simulink model "final"  (R2020b)
settings: Solver=ode4  StartTime=0.0  StopTime=10.0  FixedStep=ts  RelTol=1e-3
settings Model: Creator=auralius  LastModifiedBy=rishavgoenka
settings DataIOCC: LimitDataPoints=on  SaveFormat=Array  ReturnWorkspaceOutputs=off
settings OptimizationCC: BlockReduction=off  BooleanDataType=off  LifeSpan=inf
settings DebuggingCC: SaveWithParameterizedLinksMsg=none  UnderspecifiedInitializationDetection=Classic  MergeDetectMultiDrivingBlocksExec=none  SignalResolutionControl=TryResolveAllWithWarning  SFUnexpectedBacktrackingDiag=warning  SFNoUnconditionalDefaultTransitionDiag=warning  SFExecutionAtInitializationDiag=none  ArithmeticOperatorsInVariantConditions=warning
settings HardwareCC: ProdBitPerPointer=32  ProdBitPerSizeT=32  ProdBitPerPtrDiffT=32  ProdLargestAtomicFloat=None  ProdIntDivRoundTo=Undefined  ProdEndianess=Unspecified  ProdWordSize=32  ProdHWDeviceType=32-bit Generic  TargetUnknown=on
settings ModelReferenceCC: PropagateSignalLabelsOutOfModel=off
settings SFSimCC: SimUseLocalCustomCode=off  CustomCodeUndefinedFunction=UseInterfaceOnly
settings RTWCC: RTWUseLocalCustomCode=off
settings CodeAppCC: StateflowObjectComments=on
settings GRTTargetCC: TargetLangStandard=C89/C90 (ANSI)
settings ConfigComp: CovMetricSettings=dw  CovSaveCumulativeToWorkspaceVar=on  CovSaveSingleToWorkspaceVar=on  CovExternalEMLEnable=off

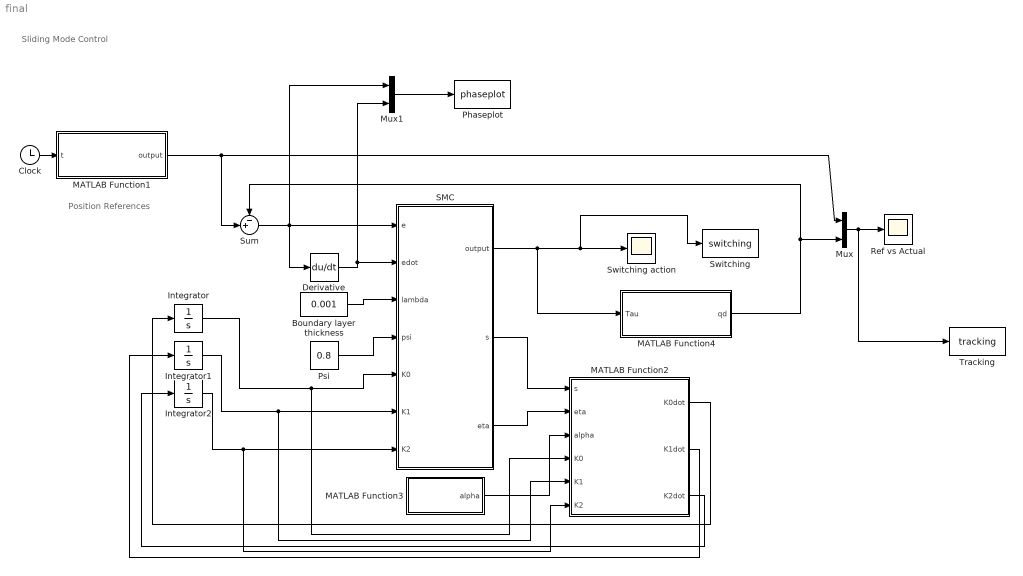
== system final ==
  note: Sliding Mode Control
  note: Position References
  Boundary layer thickness : Constant  Value=0.001
  Clock : Clock
  Derivative : Derivative
  Integrator : Integrator  InitialCondition=1
  Integrator1 : Integrator  InitialCondition=1
  Integrator2 : Integrator  InitialCondition=1
  MATLAB Function1 : MATLAB Function  TreatAsAtomicUnit=on
  MATLAB Function2 : MATLAB Function  TreatAsAtomicUnit=on
  MATLAB Function3 : MATLAB Function  TreatAsAtomicUnit=on
  MATLAB Function4 : MATLAB Function  TreatAsAtomicUnit=on
  Mux : Mux  Inputs=2
  Mux1 : Mux  Inputs=2
  Phaseplot : ToWorkspace  VariableName=phaseplot  SampleTime=-1
  Psi : Constant  Value=0.8
  Ref vs Actual : Scope
  SMC : MATLAB Function  TreatAsAtomicUnit=on
  Sum : Sum  Inputs=-+|
  Switching : ToWorkspace  VariableName=switching  SampleTime=-1
  Switching action : Scope
  Tracking : ToWorkspace  VariableName=tracking  SampleTime=-1
  wires:
  Derivative/1 -> Mux1/2, SMC/2(edot)
  Sum/1 -> Mux1/1, Derivative/1, SMC/1(e)
  Mux/1 -> Tracking/1, Ref vs Actual/1
  SMC/1(output) -> MATLAB Function4/1(Tau), Switching/1, Switching action/1
  MATLAB Function1/1(output) -> Mux/1, Sum/2
  Clock/1 -> MATLAB Function1/1(t)
  Mux1/1 -> Phaseplot/1
  SMC/2(s) -> MATLAB Function2/1(s)
  SMC/3(eta) -> MATLAB Function2/2(eta)
  MATLAB Function3/1(alpha) -> MATLAB Function2/3(alpha)
  Psi/1 -> SMC/4(psi)
  Boundary layer thickness/1 -> SMC/3(lambda)
  MATLAB Function2/1(K0dot) -> Integrator/1
  Integrator/1 -> MATLAB Function2/4(K0), SMC/5(K0)
  MATLAB Function2/2(K1dot) -> Integrator1/1
  MATLAB Function2/3(K2dot) -> Integrator2/1
  Integrator1/1 -> MATLAB Function2/5(K1), SMC/6(K1)
  Integrator2/1 -> MATLAB Function2/6(K2), SMC/7(K2)
  MATLAB Function4/1(qd) -> Sum/1, Mux/2

== matlab function final/MATLAB Function2 ==
  data: s input; K0dot output; eta input; alpha input; K0 input; K1 input; K2 input; K1dot output; K2dot output
function [K0dot, K1dot, K2dot] = gain(s, eta, alpha, K0, K1, K2)
%#codegen
    ns = norm(s);
    ne = norm(eta);
    
    K0dot = ns*(ne^0) - alpha(1)*K0;
    K1dot = ns*(ne^1) - alpha(2)*K1;
    K2dot = ns*(ne^2) - alpha(3)*K2;
end

== matlab function final/SMC ==
  data: e input; output output; edot input; lambda input; psi input; s output; eta output; K0 input; K1 input; K2 input
function [output, s, eta] = smc(e, edot, lambda, psi, K0, K1, K2)
%#codegen

    s = (psi * e + edot);
    
    eta = [e' edot']';
    
    n = norm(eta);
    
    p = K0 + K1*n + K2*n*n;
    
    output = -lambda*s - p*sign(s);

end

== matlab function final/MATLAB Function3 ==
  data: alpha output
function alpha = scalars()
%#codegen
    alpha = [2 2 2];
end

== matlab function final/MATLAB Function1 ==
  data: t input; output output
function output = generate_input(t)
%#codegen

    output = -pi/2+52.5/180*pi*(1-cos(1.26*t));
end

== matlab function final/MATLAB Function4 ==
  data: Tau input; qd output
function qd = wmr(Tau)
    % SYSTEM PARAMETERS OF WMR
    r= 0.15; % Radius of each wheel
    b= 0.75; % Wheel Base
    d= 0.30; % Forward distance of Center of mass from center of rear axle
    mc= 30.00;
    mw= 1.00;
    Ic= 15.625;
    Iw= 0.005;
    Im= 0.0025;

    m= mc+ 2*mw;

    I = Ic + 2*mw*(d^2 + b^2) + 2*Im;
    
    c= r/(2*b);
    
    phi = 0;
    
    S= [  c*(b*cos(phi)-d*sin(phi)),   c*(b*cos(phi)+d*sin(phi));
    c*(b*sin(phi) + d*cos(phi)), c*(b*sin(phi) - d*cos(phi));
                              c,                          -c;
                              1,                           0;
                              0,                           1];
    
    Nu= [4.1047, 9.2286]'; % Minimal coordinates
    Q_dot = S*Nu; % Extended coordinates
    
    om= Q_dot(3); % Phi_dot=omega
    
    Sd = [ c*om*(-b*sin(phi)-d*cos(phi)), c*om*(-b*sin(phi)+d*cos(phi));
      c*om*(b*cos(phi) - d*sin(phi)),c*om*(b*cos(phi) + d*sin(phi));
                                   0,                             0;
                                   0,                             0;
                                   0,                             0];

    M = [m, 0, 2*mw*d*sin(phi), 0 , 0;
        0, m, -2*mw*d*cos(phi), 0, 0;
        2*mw*d*sin(phi), -2*mw*d*cos(phi), I, 0, 0;
        0, 0, 0, Iw, 0;
        0, 0, 0, 0, Iw];

    C = [2*mw*d*(om^2)*cos(phi);
        2*mw*d*(om^2)*sin(phi);
        0;
        0;
        0];

    L = [0, 0;
         0, 0;
         0, 0;
         1, 0;
         0, 1];

    f2= inv(S'*M*S)*(-S'*M*Sd*Nu - S'*C);

    qd = [S*Nu; f2] + [zeros(5,2); inv(S'*M*S)*S'*L]*Tau;
end
